simulink model "Trans_2016_DIF_M2_bez_oscilograf"  (R2015a)
settings: Solver=ode23tb  StartTime=0.0  StopTime=4  FixedStep=4e-6  MaxStep=1e-5  RelTol=1e-3  AbsTol=1e-5
values from neighbouring files (symbols this model uses):
  f = 50    [matlab.mat]
  Gm = 6.28318530718e-07    [matlab.mat]
  k = k+1    (= 2)    [SIGMA_trans.m]    (also in matlab.mat = 1e-06)
  LL1 = 0.016    [matlab.mat]
  LL2 = 7.96e-06    [matlab.mat]
  Ln = 0.0060919505207    [matlab.mat]
  R1 = 3.03    [matlab.mat]
  R2 = 0.003    [matlab.mat]
  RL1 = 10    [matlab.mat]
  RL2 = 0.00125    [matlab.mat]
  Rn = 0.63798571162    [matlab.mat]
  S = 0.0216    [matlab.mat]
  w1 = 850    [matlab.mat]
  w2 = 34    [matlab.mat]
undefined symbols (not defined in the file): Lsigma, sigma1, sigma2
libraries: powerlib x77, simulink x1
(part 2 of 2)

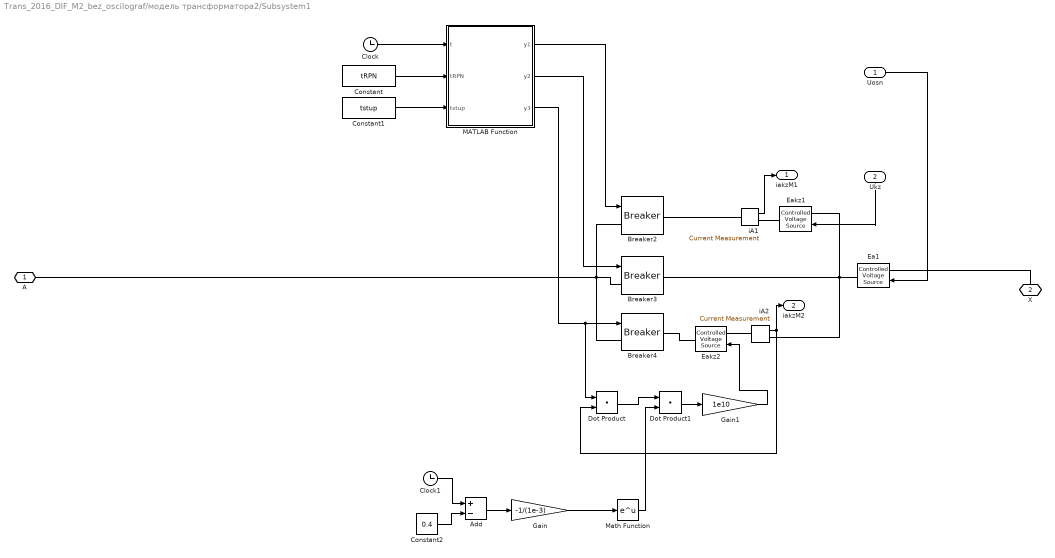
== system Trans_2016_DIF_M2_bez_oscilograf/модель трансформатора2/Subsystem1 ==
  Uosn : Inport
  Ukz : Inport  Port=2
  Add : Sum  Inputs=+-
  Breaker2 : powerlib/Elements/Breaker  InitialState=0  SwitchingTimes="[t  1e6]"  External=on  BreakerResistance=Rrpn  SnubberResistance=1e10  SnubberCapacitance=inf  Measurements=None  MoreParameters=on  NoBreakLoop=off
  Breaker3 : powerlib/Elements/Breaker  InitialState=0  SwitchingTimes="[t  1e6]"  External=on  BreakerResistance=1e-4  SnubberResistance=1e10  SnubberCapacitance=inf  Measurements=None  MoreParameters=on  NoBreakLoop=off
  Breaker4 : powerlib/Elements/Breaker  InitialState=0  SwitchingTimes="[t  1e6]"  External=on  BreakerResistance=Rrpn  SnubberResistance=1e10  SnubberCapacitance=inf  Measurements=None  MoreParameters=on  NoBreakLoop=off
  Clock : Clock
  Clock1 : Clock
  Constant : Constant  Value=tRPN
  Constant1 : Constant  Value=tstup
  Constant2 : Constant  Value=0.4
  Dot Product : DotProduct  InputSameDT=on  OutDataTypeStr=Inherit: Inherit via internal rule
  Dot Product1 : DotProduct  InputSameDT=on  OutDataTypeStr=Inherit: Inherit via internal rule
  Ea1 : powerlib/Electrical Sources/Controlled Voltage Source  Initialize=on  Source_Type=AC  Amplitude=0  Phase=0  Frequency=0  Measurements=None
  Eakz1 : powerlib/Electrical Sources/Controlled Voltage Source  Initialize=on  Source_Type=AC  Amplitude=0  Phase=0  Frequency=0  Measurements=None
  Eakz2 : powerlib/Electrical Sources/Controlled Voltage Source  Initialize=on  Source_Type=AC  Amplitude=0  Phase=0  Frequency=0  Measurements=None
  Gain : Gain  Gain=-1/(1e-3)
  Gain1 : Gain  Gain=1e10
  MATLAB Function : MATLAB Function  TreatAsAtomicUnit=on
  Math Function : Math  SaturateOnIntegerOverflow=on
  iA1 : powerlib/Measurements/Current Measurement  PhasorSimulation=off  OutputType=Complex  PSBequivalent=0
  iA2 : powerlib/Measurements/Current Measurement  PhasorSimulation=off  OutputType=Complex  PSBequivalent=0
  A : PMIOPort  Port=1  Side=Left
  X : PMIOPort  Port=2  Side=Right
  iakzM1 : Outport
  iakzM2 : Outport  Port=2
  wires:
  Gain1/1 -> Eakz2/1
  Math Function/1 -> Dot Product1/2
  Dot Product/1 -> Dot Product1/1
  Dot Product1/1 -> Gain1/1
  Gain/1 -> Math Function/1
  Add/1 -> Gain/1
  Constant2/1 -> Add/2
  Clock1/1 -> Add/1
  iA2/1 -> Dot Product/2, iakzM2/1
  iA1/1 -> iakzM1/1
  Clock/1 -> MATLAB Function/1(t)
  Constant/1 -> MATLAB Function/2(tRPN)
  Constant1/1 -> MATLAB Function/3(tstup)
  MATLAB Function/3(y3) -> Breaker4/1, Dot Product/1
  MATLAB Function/2(y2) -> Breaker3/1
  MATLAB Function/1(y1) -> Breaker2/1
  Uosn/1 -> Ea1/1
  Ukz/1 -> Eakz1/1
  connections:
  Eakz2/LConn1 -- iA2/LConn1
  Breaker2/RConn1 -- iA1/LConn1
  Breaker4/RConn1 -- Eakz2/RConn1
  iA1/RConn1 -- Eakz1/RConn1
  A/RConn1 -- Breaker4/LConn1 -- Breaker2/LConn1 -- Breaker3/LConn1
  Ea1/LConn1 -- X/RConn1
  Breaker3/RConn1 -- iA2/RConn1 -- Eakz1/LConn1 -- Ea1/RConn1

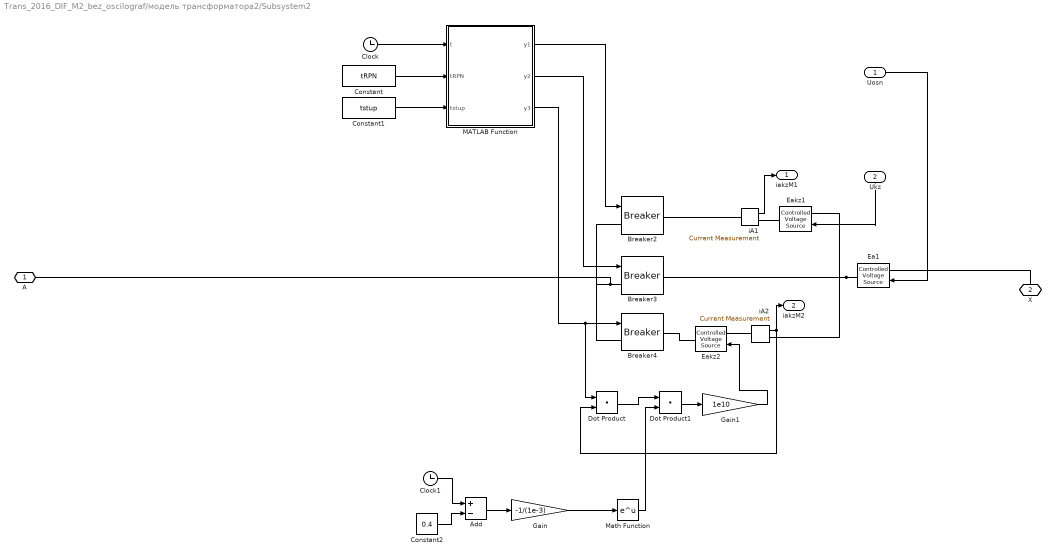
== system Trans_2016_DIF_M2_bez_oscilograf/модель трансформатора2/Subsystem2 ==
  Uosn : Inport
  Ukz : Inport  Port=2
  Add : Sum  Inputs=+-
  Breaker2 : powerlib/Elements/Breaker  InitialState=0  SwitchingTimes="[t  1e6]"  External=on  BreakerResistance=Rrpn  SnubberResistance=1e10  SnubberCapacitance=inf  Measurements=None  MoreParameters=on  NoBreakLoop=off
  Breaker3 : powerlib/Elements/Breaker  InitialState=0  SwitchingTimes="[t  1e6]"  External=on  BreakerResistance=1e-4  SnubberResistance=1e10  SnubberCapacitance=inf  Measurements=None  MoreParameters=on  NoBreakLoop=off
  Breaker4 : powerlib/Elements/Breaker  InitialState=0  SwitchingTimes="[t  1e6]"  External=on  BreakerResistance=Rrpn  SnubberResistance=1e10  SnubberCapacitance=inf  Measurements=None  MoreParameters=on  NoBreakLoop=off
  Clock : Clock
  Clock1 : Clock
  Constant : Constant  Value=tRPN
  Constant1 : Constant  Value=tstup
  Constant2 : Constant  Value=0.4
  Dot Product : DotProduct  InputSameDT=on  OutDataTypeStr=Inherit: Inherit via internal rule
  Dot Product1 : DotProduct  InputSameDT=on  OutDataTypeStr=Inherit: Inherit via internal rule
  Ea1 : powerlib/Electrical Sources/Controlled Voltage Source  Initialize=on  Source_Type=AC  Amplitude=0  Phase=0  Frequency=0  Measurements=None
  Eakz1 : powerlib/Electrical Sources/Controlled Voltage Source  Initialize=on  Source_Type=AC  Amplitude=0  Phase=0  Frequency=0  Measurements=None
  Eakz2 : powerlib/Electrical Sources/Controlled Voltage Source  Initialize=on  Source_Type=AC  Amplitude=0  Phase=0  Frequency=0  Measurements=None
  Gain : Gain  Gain=-1/(1e-3)
  Gain1 : Gain  Gain=1e10
  MATLAB Function : MATLAB Function  TreatAsAtomicUnit=on
  Math Function : Math  SaturateOnIntegerOverflow=on
  iA1 : powerlib/Measurements/Current Measurement  PhasorSimulation=off  OutputType=Complex  PSBequivalent=0
  iA2 : powerlib/Measurements/Current Measurement  PhasorSimulation=off  OutputType=Complex  PSBequivalent=0
  A : PMIOPort  Port=1  Side=Left
  X : PMIOPort  Port=2  Side=Right
  iakzM1 : Outport
  iakzM2 : Outport  Port=2
  wires:
  Ukz/1 -> Eakz1/1
  Uosn/1 -> Ea1/1
  MATLAB Function/1(y1) -> Breaker2/1
  MATLAB Function/2(y2) -> Breaker3/1
  MATLAB Function/3(y3) -> Dot Product/1, Breaker4/1
  Constant1/1 -> MATLAB Function/3(tstup)
  Constant/1 -> MATLAB Function/2(tRPN)
  Clock/1 -> MATLAB Function/1(t)
  iA1/1 -> iakzM1/1
  iA2/1 -> iakzM2/1, Dot Product/2
  Clock1/1 -> Add/1
  Constant2/1 -> Add/2
  Add/1 -> Gain/1
  Gain/1 -> Math Function/1
  Dot Product1/1 -> Gain1/1
  Dot Product/1 -> Dot Product1/1
  Math Function/1 -> Dot Product1/2
  Gain1/1 -> Eakz2/1
  connections:
  Ea1/RConn1 -- Eakz1/LConn1 -- iA2/RConn1 -- Breaker3/RConn1
  Ea1/LConn1 -- X/RConn1
  Breaker3/LConn1 -- Breaker2/LConn1 -- Breaker4/LConn1 -- A/RConn1
  iA1/RConn1 -- Eakz1/RConn1
  Breaker4/RConn1 -- Eakz2/RConn1
  Breaker2/RConn1 -- iA1/LConn1
  Eakz2/LConn1 -- iA2/LConn1

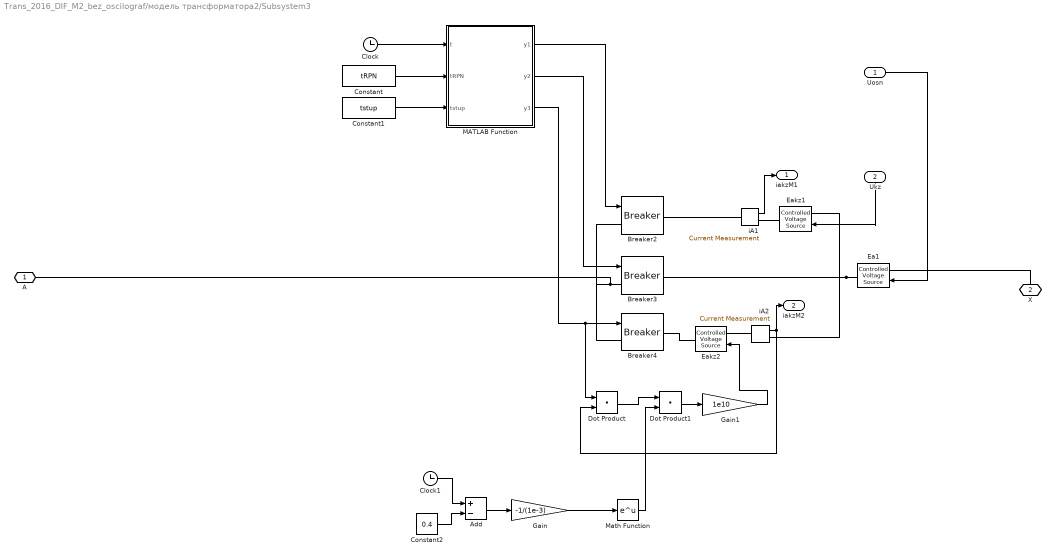
== system Trans_2016_DIF_M2_bez_oscilograf/модель трансформатора2/Subsystem3 ==
  Uosn : Inport
  Ukz : Inport  Port=2
  Add : Sum  Inputs=+-
  Breaker2 : powerlib/Elements/Breaker  InitialState=0  SwitchingTimes="[t  1e6]"  External=on  BreakerResistance=Rrpn  SnubberResistance=1e10  SnubberCapacitance=inf  Measurements=None  MoreParameters=on  NoBreakLoop=off
  Breaker3 : powerlib/Elements/Breaker  InitialState=0  SwitchingTimes="[t  1e6]"  External=on  BreakerResistance=1e-4  SnubberResistance=1e10  SnubberCapacitance=inf  Measurements=None  MoreParameters=on  NoBreakLoop=off
  Breaker4 : powerlib/Elements/Breaker  InitialState=0  SwitchingTimes="[t  1e6]"  External=on  BreakerResistance=Rrpn  SnubberResistance=1e10  SnubberCapacitance=inf  Measurements=None  MoreParameters=on  NoBreakLoop=off
  Clock : Clock
  Clock1 : Clock
  Constant : Constant  Value=tRPN
  Constant1 : Constant  Value=tstup
  Constant2 : Constant  Value=0.4
  Dot Product : DotProduct  InputSameDT=on  OutDataTypeStr=Inherit: Inherit via internal rule
  Dot Product1 : DotProduct  InputSameDT=on  OutDataTypeStr=Inherit: Inherit via internal rule
  Ea1 : powerlib/Electrical Sources/Controlled Voltage Source  Initialize=on  Source_Type=AC  Amplitude=0  Phase=0  Frequency=0  Measurements=None
  Eakz1 : powerlib/Electrical Sources/Controlled Voltage Source  Initialize=on  Source_Type=AC  Amplitude=0  Phase=0  Frequency=0  Measurements=None
  Eakz2 : powerlib/Electrical Sources/Controlled Voltage Source  Initialize=on  Source_Type=AC  Amplitude=0  Phase=0  Frequency=0  Measurements=None
  Gain : Gain  Gain=-1/(1e-3)
  Gain1 : Gain  Gain=1e10
  MATLAB Function : MATLAB Function  TreatAsAtomicUnit=on
  Math Function : Math  SaturateOnIntegerOverflow=on
  iA1 : powerlib/Measurements/Current Measurement  PhasorSimulation=off  OutputType=Complex  PSBequivalent=0
  iA2 : powerlib/Measurements/Current Measurement  PhasorSimulation=off  OutputType=Complex  PSBequivalent=0
  A : PMIOPort  Port=1  Side=Left
  X : PMIOPort  Port=2  Side=Right
  iakzM1 : Outport
  iakzM2 : Outport  Port=2
  wires:
  Ukz/1 -> Eakz1/1
  Uosn/1 -> Ea1/1
  MATLAB Function/1(y1) -> Breaker2/1
  MATLAB Function/2(y2) -> Breaker3/1
  MATLAB Function/3(y3) -> Dot Product/1, Breaker4/1
  Constant1/1 -> MATLAB Function/3(tstup)
  Constant/1 -> MATLAB Function/2(tRPN)
  Clock/1 -> MATLAB Function/1(t)
  iA1/1 -> iakzM1/1
  iA2/1 -> iakzM2/1, Dot Product/2
  Clock1/1 -> Add/1
  Constant2/1 -> Add/2
  Add/1 -> Gain/1
  Gain/1 -> Math Function/1
  Dot Product1/1 -> Gain1/1
  Dot Product/1 -> Dot Product1/1
  Math Function/1 -> Dot Product1/2
  Gain1/1 -> Eakz2/1
  connections:
  Ea1/RConn1 -- Eakz1/LConn1 -- iA2/RConn1 -- Breaker3/RConn1
  Ea1/LConn1 -- X/RConn1
  Breaker3/LConn1 -- Breaker2/LConn1 -- Breaker4/LConn1 -- A/RConn1
  iA1/RConn1 -- Eakz1/RConn1
  Breaker4/RConn1 -- Eakz2/RConn1
  Breaker2/RConn1 -- iA1/LConn1
  Eakz2/LConn1 -- iA2/LConn1

== system Trans_2016_DIF_M2_bez_oscilograf/модель трансформатора2/faz_napr ==
  "U2 " : Inport
  Demux : Demux  Outputs=3
  Ua : Outport
  Ub : Outport  Port=2
  Uc : Outport  Port=3
  wires:
  Demux/2 -> Ub/1
  Demux/1 -> Ua/1
  "U2 "/1 -> Demux/1
  Demux/3 -> Uc/1

== system Trans_2016_DIF_M2_bez_oscilograf/модель трансформатора2/faz_napr  ==
  "U1 " : Inport
  Demux : Demux  Outputs=3
  Ua : Outport
  Ub : Outport  Port=2
  Uc : Outport  Port=3
  wires:
  Demux/3 -> Uc/1
  "U1 "/1 -> Demux/1
  Demux/1 -> Ua/1
  Demux/2 -> Ub/1

== system Trans_2016_DIF_M2_bez_oscilograf/модель трансформатора2/faz_napr 1 ==
  "UvKZ " : Inport
  Demux : Demux  Outputs=3
  Ua : Outport
  Ub : Outport  Port=2
  Uc : Outport  Port=3
  wires:
  Demux/2 -> Ub/1
  Demux/1 -> Ua/1
  "UvKZ "/1 -> Demux/1
  Demux/3 -> Uc/1

== system Trans_2016_DIF_M2_bez_oscilograf/модель трансформатора2/form_matrix_C  ==
  Clock : Clock
  Constant1 : Constant  Value=tRPN
  Constant2 : Constant  Value=w1_posle
  Constant3 : Constant  Value=w2_posle
  Constant4 : Constant  Value=w2_do
  Constant5 : Constant  Value=tstup
  Constant9 : Constant  Value=w1_do
  MATLAB Function : MATLAB Function  TreatAsAtomicUnit=on
  C : Outport
  wires:
  Constant3/1 -> MATLAB Function/4(w2_posle)
  Constant2/1 -> MATLAB Function/3(w1_posle)
  Constant1/1 -> MATLAB Function/6(tRPN)
  Constant4/1 -> MATLAB Function/2(w2_do)
  Constant9/1 -> MATLAB Function/1(w1_do)
  MATLAB Function/1(C) -> C/1
  Clock/1 -> MATLAB Function/5(t)
  Constant5/1 -> MATLAB Function/7(tstup)

== system Trans_2016_DIF_M2_bez_oscilograf/модель трансформатора2/form_matrix_di ==
  di2 : Inport
  "di1 " : Inport  Port=2
  div : Inport  Port=3
  Mux : Mux  Inputs=3
      settings: DisplayOption=signals
  di : Outport
  wires:
  di2/1 -> Mux/2
  "di1 "/1 -> Mux/1
  Mux/1 -> di/1
  div/1 -> Mux/3

== system Trans_2016_DIF_M2_bez_oscilograf/модель трансформатора2/form_matrix_i ==
  i2 : Inport
  "i1 " : Inport  Port=2
  iv : Inport  Port=3
  Mux : Mux  Inputs=3
      settings: DisplayOption=signals
  i : Outport
  wires:
  "i1 "/1 -> Mux/1
  i2/1 -> Mux/2
  Mux/1 -> i/1
  iv/1 -> Mux/3

== system Trans_2016_DIF_M2_bez_oscilograf/модель трансформатора2/napr_perv_and_vtor ==
  U : Inport
  Demux : Demux  Outputs=9
  Mux : Mux  Inputs=3
      settings: DisplayOption=signals
  Mux1 : Mux  Inputs=3
      settings: DisplayOption=signals
  Mux2 : Mux  Inputs=3
      settings: DisplayOption=signals
  U2 : Outport
  URPN : Outport  Port=2
  U1 : Outport  Port=3
  wires:
  Demux/6 -> Mux1/3
  Mux1/1 -> U2/1
  Demux/4 -> Mux1/1
  Demux/5 -> Mux1/2
  Mux/1 -> U1/1
  Demux/3 -> Mux/3
  Demux/1 -> Mux/1
  Demux/2 -> Mux/2
  U/1 -> Demux/1
  Demux/7 -> Mux2/1
  Demux/8 -> Mux2/2
  Demux/9 -> Mux2/3
  Mux2/1 -> URPN/1

== system Trans_2016_DIF_M2_bez_oscilograf/модель трансформатора2/potoki ==
  "potoki " : Inport
  Demux : Demux
  potok_A : Outport
  potok_B : Outport  Port=2
  potok_C : Outport  Port=3
  potok_0 : Outport  Port=4
  wires:
  Demux/2 -> potok_B/1
  Demux/1 -> potok_A/1
  "potoki "/1 -> Demux/1
  Demux/3 -> potok_C/1
  Demux/4 -> potok_0/1

== system Trans_2016_DIF_M2_bez_oscilograf/модель трансформатора2/proizvod_kz ==
  ia : Inport
  ib : Inport  Port=2
  ic : Inport  Port=3
  Mux : Mux  Inputs=3
      settings: DisplayOption=signals
  реал. диф. блок : Subsystem  mask{k=k}
      mask prompts: k "коэффициент К"
  реал. диф. блок1 : Subsystem  mask{k=k}
      mask prompts: k "коэффициент К"
  реал. диф. блок2 : Subsystem  mask{k=k}
      mask prompts: k "коэффициент К"
  di_kz : Outport
  wires:
  ic/1 -> реал. диф. блок2/1(x)
  ib/1 -> реал. диф. блок1/1(x)
  ia/1 -> реал. диф. блок/1(x)
  реал. диф. блок/1(x') -> Mux/1
  реал. диф. блок1/1(x') -> Mux/2
  реал. диф. блок2/1(x') -> Mux/3
  Mux/1 -> di_kz/1

== system Trans_2016_DIF_M2_bez_oscilograf/модель трансформатора2/proizvod_perv ==
  ia : Inport
  ib : Inport  Port=2
  ic : Inport  Port=3
  Mux : Mux  Inputs=3
      settings: DisplayOption=signals
  реал. диф. блок : Subsystem  mask{k=k}
      mask prompts: k "коэффициент К"
  реал. диф. блок1 : Subsystem  mask{k=k}
      mask prompts: k "коэффициент К"
  реал. диф. блок2 : Subsystem  mask{k=k}
      mask prompts: k "коэффициент К"
  di_1 : Outport
  wires:
  Mux/1 -> di_1/1
  реал. диф. блок2/1(x') -> Mux/3
  реал. диф. блок1/1(x') -> Mux/2
  реал. диф. блок/1(x') -> Mux/1
  ia/1 -> реал. диф. блок/1(x)
  ib/1 -> реал. диф. блок1/1(x)
  ic/1 -> реал. диф. блок2/1(x)

== system Trans_2016_DIF_M2_bez_oscilograf/модель трансформатора2/proizvod_vtor ==
  ia : Inport
  ib : Inport  Port=2
  ic : Inport  Port=3
  Mux : Mux  Inputs=3
      settings: DisplayOption=signals
  реал. диф. блок : Subsystem  mask{k=k}
      mask prompts: k "коэффициент К"
  реал. диф. блок1 : Subsystem  mask{k=k}
      mask prompts: k "коэффициент К"
  реал. диф. блок2 : Subsystem  mask{k=k}
      mask prompts: k "коэффициент К"
  di_2 : Outport
  wires:
  Mux/1 -> di_2/1
  реал. диф. блок/1(x') -> Mux/1
  реал. диф. блок1/1(x') -> Mux/2
  реал. диф. блок2/1(x') -> Mux/3
  ic/1 -> реал. диф. блок2/1(x)
  ib/1 -> реал. диф. блок1/1(x)
  ia/1 -> реал. диф. блок/1(x)

== system Trans_2016_DIF_M2_bez_oscilograf/модель трансформатора2/toki_kz ==
  ia : Inport
  ib : Inport  Port=2
  ic : Inport  Port=3
  Mux : Mux  Inputs=3
      settings: DisplayOption=signals
  i_kz : Outport
  wires:
  Mux/1 -> i_kz/1
  ia/1 -> Mux/1
  ib/1 -> Mux/2
  ic/1 -> Mux/3

== system Trans_2016_DIF_M2_bez_oscilograf/модель трансформатора2/toki_perv ==
  ia : Inport
  ib : Inport  Port=2
  ic : Inport  Port=3
  Mux : Mux  Inputs=3
      settings: DisplayOption=signals
  i_1 : Outport
  wires:
  Mux/1 -> i_1/1
  ia/1 -> Mux/1
  ib/1 -> Mux/2
  ic/1 -> Mux/3

== system Trans_2016_DIF_M2_bez_oscilograf/модель трансформатора2/toki_vtor1 ==
  ia : Inport
  ib : Inport  Port=2
  ic : Inport  Port=3
  Mux : Mux  Inputs=3
      settings: DisplayOption=signals
  i_2 : Outport
  wires:
  Mux/1 -> i_2/1
  ia/1 -> Mux/1
  ib/1 -> Mux/2
  ic/1 -> Mux/3

== system Trans_2016_DIF_M2_bez_oscilograf/модель трансформатора2/proizvod_kz/реал. диф. блок ==
  x : Inport
  Transfer Fcn : TransferFcn  Numerator=[1 0]  Denominator=[k 1]
  x' : Outport
  wires:
  Transfer Fcn/1 -> x'/1
  x/1 -> Transfer Fcn/1

== system Trans_2016_DIF_M2_bez_oscilograf/модель трансформатора2/proizvod_kz/реал. диф. блок1 ==
  x : Inport
  Transfer Fcn : TransferFcn  Numerator=[1 0]  Denominator=[k 1]
  x' : Outport
  wires:
  x/1 -> Transfer Fcn/1
  Transfer Fcn/1 -> x'/1

== system Trans_2016_DIF_M2_bez_oscilograf/модель трансформатора2/proizvod_kz/реал. диф. блок2 ==
  x : Inport
  Transfer Fcn : TransferFcn  Numerator=[1 0]  Denominator=[k 1]
  x' : Outport
  wires:
  Transfer Fcn/1 -> x'/1
  x/1 -> Transfer Fcn/1

== system Trans_2016_DIF_M2_bez_oscilograf/модель трансформатора2/proizvod_perv/реал. диф. блок ==
  x : Inport
  Transfer Fcn : TransferFcn  Numerator=[1 0]  Denominator=[k 1]
  x' : Outport
  wires:
  x/1 -> Transfer Fcn/1
  Transfer Fcn/1 -> x'/1

== system Trans_2016_DIF_M2_bez_oscilograf/модель трансформатора2/proizvod_perv/реал. диф. блок1 ==
  x : Inport
  Transfer Fcn : TransferFcn  Numerator=[1 0]  Denominator=[k 1]
  x' : Outport
  wires:
  Transfer Fcn/1 -> x'/1
  x/1 -> Transfer Fcn/1

== system Trans_2016_DIF_M2_bez_oscilograf/модель трансформатора2/proizvod_perv/реал. диф. блок2 ==
  x : Inport
  Transfer Fcn : TransferFcn  Numerator=[1 0]  Denominator=[k 1]
  x' : Outport
  wires:
  x/1 -> Transfer Fcn/1
  Transfer Fcn/1 -> x'/1

== system Trans_2016_DIF_M2_bez_oscilograf/модель трансформатора2/proizvod_vtor/реал. диф. блок ==
  x : Inport
  Transfer Fcn : TransferFcn  Numerator=[1 0]  Denominator=[k 1]
  x' : Outport
  wires:
  x/1 -> Transfer Fcn/1
  Transfer Fcn/1 -> x'/1

== system Trans_2016_DIF_M2_bez_oscilograf/модель трансформатора2/proizvod_vtor/реал. диф. блок1 ==
  x : Inport
  Transfer Fcn : TransferFcn  Numerator=[1 0]  Denominator=[k 1]
  x' : Outport
  wires:
  Transfer Fcn/1 -> x'/1
  x/1 -> Transfer Fcn/1

== system Trans_2016_DIF_M2_bez_oscilograf/модель трансформатора2/proizvod_vtor/реал. диф. блок2 ==
  x : Inport
  Transfer Fcn : TransferFcn  Numerator=[1 0]  Denominator=[k 1]
  x' : Outport
  wires:
  x/1 -> Transfer Fcn/1
  Transfer Fcn/1 -> x'/1

== matlab function Trans_2016_DIF_M2_bez_oscilograf/модель трансформатора2/Form_Lsigma/MATLAB Function ==
  data: LsigmaX input; Lsigma output; C input; w1 input; w2 input
function Lsigma = Lsigma_form(LsigmaX,C,w1,w2)
%#codegen

Lsigma = zeros(9);
Lsigma(1,1)=LsigmaX(1,1)*(C(1,1)/w1);
Lsigma(2,2)=LsigmaX(2,2)*(C(2,2)/w1);
Lsigma(3,3)=LsigmaX(3,3)*(C(3,3)/w1);
Lsigma(4,4)=LsigmaX(4,4)*abs((C(1,4)/w2));
Lsigma(5,5)=LsigmaX(5,5)*abs((C(2,5)/w2));
Lsigma(6,6)=LsigmaX(6,6)*abs((C(3,6)/w2));
Lsigma(7,7)=LsigmaX(1,1)*abs((C(1,7)/w1));
Lsigma(8,8)=LsigmaX(2,2)*abs((C(2,8)/w1));
Lsigma(9,9)=LsigmaX(3,3)*abs((C(3,9)/w1));

== matlab function Trans_2016_DIF_M2_bez_oscilograf/модель трансформатора2/Subsystem2/MATLAB Function ==
  data: t input; tRPN input; y1 output; tstup input; y2 output; y3 output
function [y1,y2,y3]= fcn(t,tRPN,tstup)
%#codegen

y1=0;
y2=1;
y3=0;

%# до срабатывания РПН только центральный провод
if t<tRPN
    y1=0;
    y2=1;
    y3=0;
end;
%# центральный отключился, подключился вместо него провод с резистором
if (t>tRPN)&& (t<tRPN+tstup)
    y1=1;
    y2=0;
    y3=0;
end;
%# замкнулся второй контакт с резистором на других витках
if (t>tRPN+tstup)&& (t<tRPN+2*tstup)
    y1=1;
    y2=0;
    y3=1;
end;
%# первый контакт с резисторами разомкнулся
if (t>tRPN+2*tstup)&& (t<tRPN+3*tstup)
    y1=0;
    y2=0;
    y3=1;
end;
%# замкнулся центральный (только он)
if (t>(tRPN+3*tstup))
    y1=0;
    y2=1;
    y3=0;
end;

== matlab function Trans_2016_DIF_M2_bez_oscilograf/модель трансформатора2/Subsystem1/MATLAB Function ==
  data: t input; tRPN input; y1 output; tstup input; y2 output; y3 output
function [y1,y2,y3]= fcn(t,tRPN,tstup)
%#codegen

y1=0;
y2=1;
y3=0;

%# до срабатывания РПН только центральный провод
if t<tRPN
    y1=0;
    y2=1;
    y3=0;
end;
%# центральный отключился, подключился вместо него провод с резистором
if (t>tRPN)&& (t<tRPN+tstup)
    y1=1;
    y2=0;
    y3=0;
end;
%# замкнулся второй контакт с резистором на других витках
if (t>tRPN+tstup)&& (t<tRPN+2*tstup)
    y1=1;
    y2=0;
    y3=1;
end;
%# первый контакт с резисторами разомкнулся
if (t>tRPN+2*tstup)&& (t<tRPN+3*tstup)
    y1=0;
    y2=0;
    y3=1;
end;
%# замкнулся центральный (только он)
if (t>(tRPN+3*tstup))
    y1=0;
    y2=1;
    y3=0;
end;

== matlab function Trans_2016_DIF_M2_bez_oscilograf/модель трансформатора2/Subsystem3/MATLAB Function ==
  data: t input; tRPN input; y1 output; tstup input; y2 output; y3 output
function [y1,y2,y3]= fcn(t,tRPN,tstup)
%#codegen

y1=0;
y2=1;
y3=0;

%# до срабатывания РПН только центральный провод
if t<tRPN
    y1=0;
    y2=1;
    y3=0;
end;
%# центральный отключился, подключился вместо него провод с резистором
if (t>tRPN)&& (t<tRPN+tstup)
    y1=1;
    y2=0;
    y3=0;
end;
%# замкнулся второй контакт с резистором на других витках
if (t>tRPN+tstup)&& (t<tRPN+2*tstup)
    y1=1;
    y2=0;
    y3=1;
end;
%# первый контакт с резисторами разомкнулся
if (t>tRPN+2*tstup)&& (t<tRPN+3*tstup)
    y1=0;
    y2=0;
    y3=1;
end;
%# замкнулся центральный (только он)
if (t>(tRPN+3*tstup))
    y1=0;
    y2=1;
    y3=0;
end;

== matlab function Trans_2016_DIF_M2_bez_oscilograf/модель трансформатора2/form_matrix_C /MATLAB Function ==
  data: C output; w1_do input; w2_do input; w1_posle input; w2_posle input; t input; tRPN input; tstup input
function C = Matrix_C(w1_do,w2_do,w1_posle,w2_posle,t,tRPN,tstup)
%#создание матрицы С
%# до срабатывания РПН только центральный провод
C = [w1_do(1) 0 0 -w2_do(1) 0 0 0 0 0;0 w1_do(2) 0 0 -w2_do(2) 0 0 0 0; 0 0 w1_do(3) 0 0 -w2_do(3) 0 0 0;0 0 0 0 0 0 0 0 0];
%# центральный отключился, подключился вместо него провод с резистором
if (t>tRPN)&& (t<tRPN+tstup)
   C = [w1_do(1) 0 0 -w2_posle(1) 0 0 0 0 0;0 w1_do(2) 0 0 -w2_posle(2) 0 0 0 0; 0 0 w1_do(3) 0 0 -w2_posle(3) 0 0 0;0 0 0 0 0 0 0 0 0]; 
end;
%# замкнулся второй контакт с резистором на других витках
if (t>tRPN+tstup)&& (t<tRPN+2*tstup)
   C = [w1_posle(1) 0 0 -w2_posle(1) 0 0 (w1_do(1)-w1_posle(1)) 0 0;0 w1_posle(2) 0 0 -w2_posle(2) 0 0 (w1_do(2)-w1_posle(2)) 0; 0 0 w1_posle(3) 0 0 -w2_posle(3) 0 0 (w1_do(3)-w1_posle(3));0 0 0 0 0 0 0 0 0]; 
end;
%# первый контакт с резисторами разомкнулся
if (t>tRPN+2*tstup)&& (t<tRPN+3*tstup)
   C = [w1_posle(1) 0 0 -w2_posle(1) 0 0 0 0 0;0 w1_posle(2) 0 0 -w2_posle(2) 0 0 0 0; 0 0 w1_posle(3) 0 0 -w2_posle(3) 0 0 0;0 0 0 0 0 0 0 0 0]; 
end;
%# замкнулся центральный (только он)
if (t>tRPN+3*tstup)
   C = [w1_posle(1) 0 0 -w2_posle(1) 0 0 0 0 0;0 w1_posle(2) 0 0 -w2_posle(2) 0 0 0 0; 0 0 w1_posle(3) 0 0 -w2_posle(3) 0 0 0;0 0 0 0 0 0 0 0 0]; 
end;

== matlab function Trans_2016_DIF_M2_bez_oscilograf/Subsystem1/Subsystem4/MATLAB Function ==
  data: t input; y output; T_period input; x input; x_pred input; y_pred input
function y = fcn(t,T_period,x,x_pred,y_pred)
%#задание начального значения
y=0;
if (x_pred>x) && (x_pred>0)&& (x<=0)
   dt=mod(t,T_period);
   y=dt*360/T_period;
else
    y=y_pred;
end;

== matlab function Trans_2016_DIF_M2_bez_oscilograf/Subsystem2/Subsystem4/MATLAB Function ==
  data: t input; y output; T_period input; x input; x_pred input; y_pred input
function y = fcn(t,T_period,x,x_pred,y_pred)
%#задание начального значения
y=0;
if (x_pred>x) && (x_pred>0)&& (x<=0)
   dt=mod(t,T_period);
   y=dt*360/T_period;
else
    y=y_pred;
end;

== matlab function Trans_2016_DIF_M2_bez_oscilograf/Subsystem3/Subsystem4/MATLAB Function ==
  data: t input; y output; T_period input; x input; x_pred input; y_pred input
function y = fcn(t,T_period,x,x_pred,y_pred)
%#задание начального значения
y=0;
if (x_pred>x) && (x_pred>0)&& (x<=0)
   dt=mod(t,T_period);
   y=dt*360/T_period;
else
    y=y_pred;
end;

== matlab function Trans_2016_DIF_M2_bez_oscilograf/Subsystem4/Subsystem4/MATLAB Function ==
  data: t input; y output; T_period input; x input; x_pred input; y_pred input
function y = fcn(t,T_period,x,x_pred,y_pred)
%#задание начального значения
y=0;
if (x_pred>x) && (x_pred>0)&& (x<=0)
   dt=mod(t,T_period);
   y=dt*360/T_period;
else
    y=y_pred;
end;

== matlab function Trans_2016_DIF_M2_bez_oscilograf/Subsystem7/Subsystem4/MATLAB Function ==
  data: t input; y output; T_period input; x input; x_pred input; y_pred input
function y = fcn(t,T_period,x,x_pred,y_pred)
%#задание начального значения
y=0;
if (x_pred>x) && (x_pred>0)&& (x<=0)
   dt=mod(t,T_period);
   y=dt*360/T_period;
else
    y=y_pred;
end;

== matlab function Trans_2016_DIF_M2_bez_oscilograf/Subsystem5/Subsystem4/MATLAB Function ==
  data: t input; y output; T_period input; x input; x_pred input; y_pred input
function y = fcn(t,T_period,x,x_pred,y_pred)
%#задание начального значения
y=0;
if (x_pred>x) && (x_pred>0)&& (x<=0)
   dt=mod(t,T_period);
   y=dt*360/T_period;
else
    y=y_pred;
end;

== matlab function Trans_2016_DIF_M2_bez_oscilograf/Subsystem6/Subsystem4/MATLAB Function ==
  data: t input; y output; T_period input; x input; x_pred input; y_pred input
function y = fcn(t,T_period,x,x_pred,y_pred)
%#задание начального значения
y=0;
if (x_pred>x) && (x_pred>0)&& (x<=0)
   dt=mod(t,T_period);
   y=dt*360/T_period;
else
    y=y_pred;
end;

== matlab function Trans_2016_DIF_M2_bez_oscilograf/Subsystem8/Subsystem4/MATLAB Function ==
  data: t input; y output; T_period input; x input; x_pred input; y_pred input
function y = fcn(t,T_period,x,x_pred,y_pred)
%#задание начального значения
y=0;
if (x_pred>x) && (x_pred>0)&& (x<=0)
   dt=mod(t,T_period);
   y=dt*360/T_period;
else
    y=y_pred;
end;

== matlab function Trans_2016_DIF_M2_bez_oscilograf/Subsystem9/Subsystem4/MATLAB Function ==
  data: t input; y output; T_period input; x input; x_pred input; y_pred input
function y = fcn(t,T_period,x,x_pred,y_pred)
%#задание начального значения
y=0;
if (x_pred>x) && (x_pred>0)&& (x<=0)
   dt=mod(t,T_period);
   y=dt*360/T_period;
else
    y=y_pred;
end;

== matlab function Trans_2016_DIF_M2_bez_oscilograf/Subsystem10/Subsystem4/MATLAB Function ==
  data: t input; y output; T_period input; x input; x_pred input; y_pred input
function y = fcn(t,T_period,x,x_pred,y_pred)
%#задание начального значения
y=0;
if (x_pred>x) && (x_pred>0)&& (x<=0)
   dt=mod(t,T_period);
   y=dt*360/T_period;
else
    y=y_pred;
end;

== matlab function Trans_2016_DIF_M2_bez_oscilograf/модель трансформатора2/трансформатор трёхстержневой ==
  data: t input; Gm input; Lsigmavx input; C input; ii input; di input; U output; sigma1 input; sigma2 input; POTOKI output; Lbb output; izmRprov input
function [U,POTOKI,Lbb]= DifL(t,Gm,Lsigmavx,C,ii,di,sigma1,sigma2,izmRprov)

K1=0;
if t==0.01
    K1=K1;
end;

%# так как до этого была строка, а нужен столбец
ii=ii';
di=di';


%# зададим матрицу А и Lsigma
A = [-1 -1 -1 1];
Lsigma = Lsigmavx;
%#присвоение начальных значений матрицам J (около 0)
J01=sigma1(4,1);
J02=sigma2(4,1);
J = [J01; J02; J01; 0];
F=C*ii';
%#присвоение начальных значений матрицам LL (около 0)
L01=sigma1(3,1);
L02=sigma2(3,1);
LL= [L01 0 0 0;0 L02 0 0; 0 0 L01 0; 0 0 0 Gm];

%# колличество элементов в масиве
K1=0; %# количество попыток рандомным методом
k=1; zzz=0;
usl = 1;
POTOK = [0; 0; 0; 0];
NUMB = [1 1 1] ;
NUMB_pred= NUMB;

while usl
  %# ' - транспонирование
Ysigma = A*LL*(A');
Isigma = -A*(LL*F+J);
%# inv - обратная матрица inv ( A) * B с A \ B
fix= (inv(Ysigma))*Isigma;
%# Находим новые значения потенциалов 
Up= (A')*fix;
%# Находим новые значения потоков U с плюсом, так как - уже есть в формуле выше 
POTOK =LL*Up+LL*F+J;


%# колличество элементов в масиве
D=length(sigma1);
%# для первой ветви
perv = 1;
if (abs(POTOK(1))>sigma1(1,D-1))
   %# пересчёт 
  LL(1,1)= sigma1(3,D);
  J(1)=sigma1(4,D);
  NUMB(1)= D;
else 
      for i=1:1:(D-1)
        if (abs(POTOK(1))<sigma1(1,i) && perv)
            %# пересчёт 
          LL(1,1)= sigma1(3,i);
          J(1)=sigma1(4,i);
          perv = 0;
          NUMB(1)= i;
        end;
       end;   
end;
if (POTOK(1)<0)
   J(1)=-J(1);
   NUMB(1)=-NUMB(1);
end;
 

%# колличество элементов в масиве
D=length(sigma2);
%# для второй ветви
perv = 1;
if (abs(POTOK(2))>sigma2(1,D-1))
   %# пересчёт 
  LL(2,2)= sigma2(3,D);
  J(2)=sigma2(4,D);
  NUMB(2)= D;
else 
      for i=1:1:(D-1)
        if (abs(POTOK(2))<sigma2(1,i) && perv)
            %# пересчёт 
          LL(2,2)= sigma2(3,i);
          J(2)=sigma2(4,i);
          perv = 0;
          NUMB(2)= i;
        end;
       end;   
end;
if (POTOK(2)<0)
   J(2)=-J(2);
   NUMB(2)=-NUMB(2);
end;
 

%# колличество элементов в масиве
D=length(sigma1);
%# для третьей ветви
perv = 1;
if (abs(POTOK(3))>sigma1(1,D-1))
   %# пересчёт 
  LL(3,3)= sigma1(3,D);
  J(3)=sigma1(4,D);
  NUMB(3)= D;
else 
      for i=1:1:(D-1)
        if (abs(POTOK(3))<sigma1(1,i) && perv)
            %# пересчёт 
          LL(3,3)= sigma1(3,i);
          J(3)=sigma1(4,i);
          perv = 0;
          NUMB(3)= i;
        end;
       end;   
end;
if (POTOK(3)<0)
   J(3)=-J(3);
   NUMB(3)=-NUMB(3);
end;




%# рандомный метод (если не сходится)
if k==39
    for i=1:1:3
         NUMB(i)=NovIndex(D);
         l=1;
         if i==2;
             l=2;
         end;
         if i ~= 2;
             l=1;
         end;
         
         if NUMB(i)>0
             if l==1
                 LL(i,i)= sigma1(3,NUMB(i));
                 J(i)=sigma1(4,NUMB(i));
             else
                 LL(i,i)= sigma2(3,NUMB(i));
                 J(i)=sigma2(4,NUMB(i));
             end;
         else
             if l==1
                 LL(i,i)= sigma1(3,-NUMB(i));
                 J(i)=-sigma1(4,-NUMB(i));
             else
                 LL(i,i)= sigma2(3,-NUMB(i));
                 J(i)=-sigma2(4,-NUMB(i));
             end;
         end;
    end;
    k=0;
    K1=K1+1;
end;


%# выход из цикла
for i=1:1:3
    if (NUMB_pred(i) == NUMB(i))
       zzz=zzz+1;
    end;
end;
 
if (zzz==3)
  usl = 0;
end;
zzz=0;
k=k+1; 
NUMB_pred = NUMB;
end;
 
 
LM=(C')*LL*C+Lsigma;
LLu=A*LL*(A');
 
%# Итоговый расчёт
LBB= LM -  (C')*LL*(A')*(inv(LLu))*A*LL*C;

Ue=LBB*di';

%# учёт изменения сопротивления проводов от изменения числа витков
%#izmRprov(1) = R1
%#izmRprov(2) = w1
Ue(1) =Ue(1)+ii(1)*(izmRprov(1)*C(1,1)/izmRprov(2)-izmRprov(1));
Ue(2) =Ue(2)+ii(2)*(izmRprov(1)*C(2,2)/izmRprov(2)-izmRprov(1));
Ue(3) =Ue(3)+ii(3)*(izmRprov(1)*C(3,3)/izmRprov(2)-izmRprov(1));

POTOKI=POTOK;



    U=Ue;

Lbb=LBB;

%#  round(X) округление 
%# rand рандомно одно число
function y = NovIndex(D)
usl_1=1;
z=0;
while usl_1
   z=round(D*rand);
   if z~=0    % ~= не равно
      usl_1= 0; 
   end;
end;
if rand<0.5
    z=-z;
end;
y=z;

== matlab function Trans_2016_DIF_M2_bez_oscilograf/Subsystem16/Subsystem4/MATLAB Function ==
  data: t input; y output; T_period input; x input; x_pred input; y_pred input
function y = fcn(t,T_period,x,x_pred,y_pred)
%#задание начального значения
y=0;
if (x_pred>x) && (x_pred>0)&& (x<=0)
   dt=mod(t,T_period);
   y=dt*360/T_period;
else
    y=y_pred;
end;

== matlab function Trans_2016_DIF_M2_bez_oscilograf/Subsystem17/Subsystem4/MATLAB Function ==
  data: t input; y output; T_period input; x input; x_pred input; y_pred input
function y = fcn(t,T_period,x,x_pred,y_pred)
%#задание начального значения
y=0;
if (x_pred>x) && (x_pred>0)&& (x<=0)
   dt=mod(t,T_period);
   y=dt*360/T_period;
else
    y=y_pred;
end;

== matlab function Trans_2016_DIF_M2_bez_oscilograf/Subsystem18/Subsystem4/MATLAB Function ==
  data: t input; y output; T_period input; x input; x_pred input; y_pred input
function y = fcn(t,T_period,x,x_pred,y_pred)
%#задание начального значения
y=0;
if (x_pred>x) && (x_pred>0)&& (x<=0)
   dt=mod(t,T_period);
   y=dt*360/T_period;
else
    y=y_pred;
end;
